simulink model "simulate"  (Simulink 9.2)
settings: Solver=ode4  StartTime=0  StopTime=30  FixedStep=0.001  RelTol=1e-3
settings Model: Creator=lenovo  LastModifiedBy=lenovo  ExtModeTrigMode=oneshot  ExtModeArmWhenConnect=off
settings SolverCC: ZeroCrossControl=DisableAll
settings DataIOCC: LimitDataPoints=off  SignalLoggingName=sigsOut
settings OptimizationCC: BooleanDataType=off  LifeSpan=auto
settings DebuggingCC: AlgebraicLoopMsg=none  ArtificialAlgebraicLoopMsg=none  SaveWithParameterizedLinksMsg=none  SignalResolutionControl=TryResolveAllWithWarning  MultiTaskDSMMsg=warning  MultiTaskCondExecSysMsg=none  FcnCallInpInsideContextMsg=error  StateNameClashWarn=none  SFUnexpectedBacktrackingDiag=error  SFNoUnconditionalDefaultTransitionDiag=error  SFExecutionAtInitializationDiag=warning
settings HardwareCC: TargetBitPerPointer=64  TargetBitPerSizeT=64  TargetBitPerPtrDiffT=64  TargetLongLongMode=on  TargetIntDivRoundTo=Zero  TargetEndianess=LittleEndian  TargetWordSize=64  TargetHWDeviceType=MATLAB Host  ProdEqTarget=off
settings SFSimCC: SimUseLocalCustomCode=on
settings RTWCC: RTWUseLocalCustomCode=on
settings CodeAppCC: StateflowObjectComments=off
settings GRTTargetCC: TargetLangStandard=C99 (ISO)  GeneratePreprocessorConditionals=Use local settings
settings ConfigComp: CovExternalEMLEnable=on

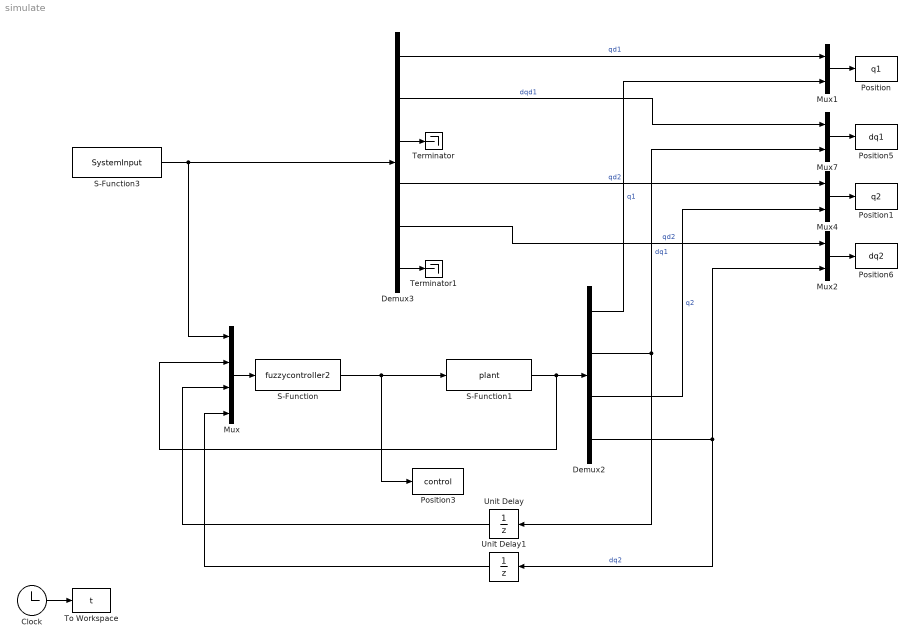
== system simulate ==
  Clock : Clock
  Demux2 : Demux
  Demux3 : Demux  Outputs=6
  Mux : Mux
  Mux{1..2,4,7} (4 alike) : Mux  Inputs=2
  Position : ToWorkspace  VariableName=q1  SampleTime=-1
  Position1 : ToWorkspace  VariableName=q2  SampleTime=-1
  Position3 : ToWorkspace  VariableName=control  SampleTime=-1
  Position5 : ToWorkspace  VariableName=dq1  SampleTime=-1
  Position6 : ToWorkspace  VariableName=dq2  SampleTime=-1
  S-Function : S-Function  FunctionName=fuzzycontroller2  SFunctionDeploymentMode=off  EnableBusSupport=off
  S-Function1 : S-Function  FunctionName=plant  SFunctionDeploymentMode=off  EnableBusSupport=off
  S-Function3 : S-Function  FunctionName=SystemInput  SFunctionDeploymentMode=off  EnableBusSupport=off
  Terminator : Terminator
  Terminator1 : Terminator
  To Workspace : ToWorkspace  VariableName=t  SampleTime=-1
  Unit Delay : UnitDelay  SampleTime=-1
  Unit Delay1 : UnitDelay  SampleTime=-1
  wires:
  Mux2/1 -> Position6/1
  S-Function3/1 -> Mux/1, Demux3/1
  Demux2/1 -> Mux1/2  "q1"
  Mux7/1 -> Position5/1
  Demux2/4 -> Mux2/2, Unit Delay1/1  "dq2"
  Demux3/2 -> Mux7/1  "dqd1"
  Demux3/1 -> Mux1/1  "qd1"
  Mux4/1 -> Position1/1
  Demux2/2 -> Mux7/2, Unit Delay/1  "dq1"
  S-Function1/1 -> Mux/2, Demux2/1
  Mux1/1 -> Position/1
  Clock/1 -> To Workspace/1
  Mux/1 -> S-Function/1
  S-Function/1 -> S-Function1/1, Position3/1
  Demux3/5 -> Mux2/1  "qd2"
  Demux3/4 -> Mux4/1  "qd2"
  Unit Delay/1 -> Mux/3
  Unit Delay1/1 -> Mux/4
  Demux2/3 -> Mux4/2  "q2"
  Demux3/3 -> Terminator/1
  Demux3/6 -> Terminator1/1
